simulink model "simulink_2D_Quadrotor_and_pendulum"  (R2023a)
settings: Solver=ode4  StartTime=0.0  StopTime=15  FixedStep=1e-3  RelTol=1e-3
values from neighbouring files (symbols this model uses):
  d = 0.1    [parametry_Lagrange.m]    (also in parametry_a_vizualizace.m)
  g = 9.81    [parametry_Lagrange.m]    (also in parametry_a_vizualizace.m)
  Ikv = 0.00025    [parametry_Lagrange.m]    (also in parametry_a_vizualizace.m)
  Ip = m*d^2    (= 0.0001)    [parametry_Lagrange.m]    (also in parametry_a_vizualizace.m)
  k = 0    [parametry_Lagrange.m]    (also in parametry_a_vizualizace.m = 0.1)
  kp = 0    [parametry_Lagrange.m]    (also in parametry_a_vizualizace.m = 0.01)
  L = 0.086    [parametry_Lagrange.m]    (also in parametry_a_vizualizace.m)
  M = 0.5    [parametry_Lagrange.m]    (also in parametry_a_vizualizace.m)
  m = 0.01    [parametry_Lagrange.m]    (also in parametry_a_vizualizace.m)
libraries: slpidlib x3, simulink_extras x2
settings Model: PacingRate=5  Creator=Admin  LastModifiedBy=Admin

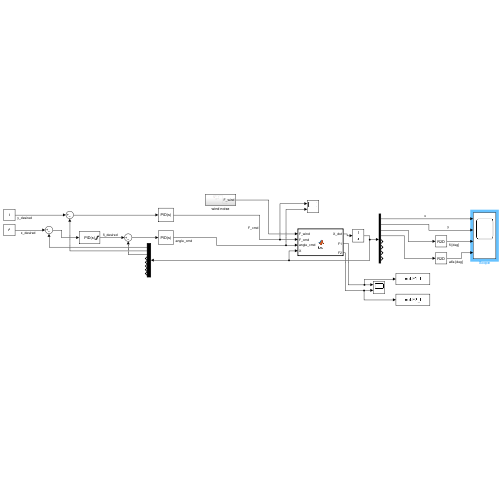
[thumbnail: Simulink's stored preview of the top-level diagram]
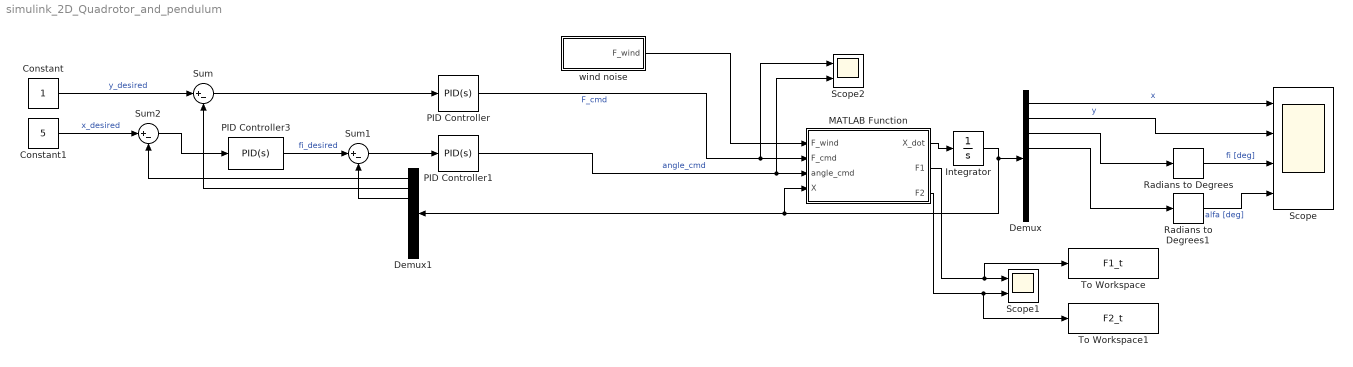
== system simulink_2D_Quadrotor_and_pendulum ==
  Constant : Constant
  Constant1 : Constant  Value=5
  Demux : Demux  Outputs=8
  Demux1 : Demux  Outputs=8
  Integrator : Integrator  InitialCondition=[0;0;0;0;0;0;0;0]  UpperSaturationLimit=[inf; inf; inf; pi; inf; inf; inf; inf]  LowerSaturationLimit=[-inf; -inf; -inf; -pi; -inf; -inf; -inf; -inf]  IgnoreLimit=on
  MATLAB Function : MATLAB Function  TreatAsAtomicUnit=on
  PID Controller : slpidlib/PID Controller  Controller=PID  Form=Parallel  TimeDomain=Continuous-time  UseExternalTs=off  SampleTime=-1  IntegratorMethod=Forward Euler  FilterMethod=Forward Euler  ControllerParametersSource=internal  P=1.05198564586534  I=0.256782152616  UseKiTs=off  D=0.957105978156924  N=439.006628920084  UseFilter=on  TunerSelectOption=Transfer Function Based (PID Tuner App)  InitialConditionSource=internal  InitialConditionForIntegrator=0  InitialConditionForFilter=0  DifferentiatorICPrevScaledInput=0  ExternalReset=none  TrackingMode=off  Kt=1  LimitOutput=off  SatLimitsSource=internal  UpperSaturationLimit=inf  LowerSaturationLimit=-inf  LinearizeAsGain=on  AntiWindupMode=none  Kb=1  LimitIntegrator=off  UpperIntegratorSaturationLimit=inf  LowerIntegratorSaturationLimit=-inf  POutMin=[]  POutMax=[]  IOutMin=[]  IOutMax=[]  DOutMin=[]  DOutMax=[]  NOutMin=[]  NOutMax=[]  SumOutMin=[]  SumOutMax=[]  SaturationOutMin=[]  SaturationOutMax=[]  PParamMin=[]  PParamMax=[]  IParamMin=[]  IParamMax=[]  DParamMin=[]  DParamMax=[]  NParamMin=[]  NParamMax=[]  KbParamMin=[]  KbParamMax=[]  KtParamMin=[]  KtParamMax=[]  KbOutMin=[]  KbOutMax=[]  KtOutMin=[]  KtOutMax=[]  IntegratorOutMin=[]  IntegratorOutMax=[]  FilterOutMin=[]  FilterOutMax=[]  SumI1OutMin=[]  SumI1OutMax=[]  SumI2OutMin=[]  SumI2OutMax=[]  SumI3OutMin=[]  SumI3OutMax=[]  SumI4OutMin=[]  SumI4OutMax=[]  SumDOutMin=[]  SumDOutMax=[]  DifferentiatorOutMin=[]  DifferentiatorOutMax=[]  FilterDiffOutCoefMin=[]  FilterDiffOutCoefMax=[]  ReciprocalOutMin=[]  ReciprocalOutMax=[]  SumDenOutMin=[]  SumDenOutMax=[]  SumNumOutMin=[]  SumNumOutMax=[]  DivideOutMin=[]  DivideOutMax=[]  UdiffTsProdOutMin=[]  UdiffTsProdOutMax=[]  NTsProdOutMin=[]  NTsProdOutMax=[]  UintegralTsProdOutMin=[]  UintegralTsProdOutMax=[]  UngainTsProdOutMin=[]  UngainTsProdOutMax=[]  ClampingZeroOutDataTypeStr=Inherit: Inherit via back propagation  ClampingZeroOutMin=[]  ClampingZeroOutMax=[]  FilterDenConstantOutDataTypeStr=Inherit: Inherit via back propagation  FilterDenConstantOutMin=[]  FilterDenConstantOutMax=[]  PCopyOutDataTypeStr=Inherit: Inherit via back propagation  PCopyOutMin=[]  PCopyOutMax=[]  NCopyOutDataTypeStr=Inherit: Inherit via back propagation  NCopyOutMin=[]  NCopyOutMax=[]  IntegratorContinuousStateAttributes=''  IntegratorStateMustResolveToSignalObject=off  IntegratorRTWStateStorageClass=Auto  FilterContinuousStateAttributes=''  FilterStateMustResolveToSignalObject=off  FilterRTWStateStorageClass=Auto  ParallelPVariant=InternalParameters  IdealPVariant=Disabled  IVariant=InternalParameters  DVariant=InternalParameters  IntegratorVariant=Continuous  SatVariant=Disabled  AWVariant=Passthrough  PCopyVariant=Disabled  TRVariant=Disabled  FdbkBlocksVariant=Forward  IdealPFdbkVariant=Disabled  SatFdbkVariant=Disabled  DerivativeFilterVariant=ContFilter  NVariant=InternalParameters  NCopyVariant=Disabled  FilterICVariant=InternalICsFilter  IntegratorICVariant=InternalICs  ExternalResetVariant=Disabled  TRSumVariant=Passthrough  SumFdbkVariant=Disabled  SumVariant=Sum_PID  TsampFilterVariant=InternalTs  TsampNgainVariant=Passthrough  TsampIntegralVariant=Passthrough  ExternalSaturationOutDataTypeStr=Inherit: Same as second input
  PID Controller1 : slpidlib/PID Controller  Controller=PID  Form=Parallel  TimeDomain=Continuous-time  UseExternalTs=off  SampleTime=-1  IntegratorMethod=Forward Euler  FilterMethod=Forward Euler  ControllerParametersSource=internal  P=0.0094983620396136  I=0.000297296508384773  UseKiTs=off  D=0.00438770568667322  N=3.63078054770101  UseFilter=on  TunerSelectOption=Transfer Function Based (PID Tuner App)  InitialConditionSource=internal  InitialConditionForIntegrator=0  InitialConditionForFilter=0  DifferentiatorICPrevScaledInput=0  ExternalReset=none  TrackingMode=off  Kt=1  LimitOutput=off  SatLimitsSource=internal  UpperSaturationLimit=inf  LowerSaturationLimit=-inf  LinearizeAsGain=on  AntiWindupMode=none  Kb=1  LimitIntegrator=off  UpperIntegratorSaturationLimit=inf  LowerIntegratorSaturationLimit=-inf  POutMin=[]  POutMax=[]  IOutMin=[]  IOutMax=[]  DOutMin=[]  DOutMax=[]  NOutMin=[]  NOutMax=[]  SumOutMin=[]  SumOutMax=[]  SaturationOutMin=[]  SaturationOutMax=[]  PParamMin=[]  PParamMax=[]  IParamMin=[]  IParamMax=[]  DParamMin=[]  DParamMax=[]  NParamMin=[]  NParamMax=[]  KbParamMin=[]  KbParamMax=[]  KtParamMin=[]  KtParamMax=[]  KbOutMin=[]  KbOutMax=[]  KtOutMin=[]  KtOutMax=[]  IntegratorOutMin=[]  IntegratorOutMax=[]  FilterOutMin=[]  FilterOutMax=[]  SumI1OutMin=[]  SumI1OutMax=[]  SumI2OutMin=[]  SumI2OutMax=[]  SumI3OutMin=[]  SumI3OutMax=[]  SumI4OutMin=[]  SumI4OutMax=[]  SumDOutMin=[]  SumDOutMax=[]  DifferentiatorOutMin=[]  DifferentiatorOutMax=[]  FilterDiffOutCoefMin=[]  FilterDiffOutCoefMax=[]  ReciprocalOutMin=[]  ReciprocalOutMax=[]  SumDenOutMin=[]  SumDenOutMax=[]  SumNumOutMin=[]  SumNumOutMax=[]  DivideOutMin=[]  DivideOutMax=[]  UdiffTsProdOutMin=[]  UdiffTsProdOutMax=[]  NTsProdOutMin=[]  NTsProdOutMax=[]  UintegralTsProdOutMin=[]  UintegralTsProdOutMax=[]  UngainTsProdOutMin=[]  UngainTsProdOutMax=[]  ClampingZeroOutDataTypeStr=Inherit: Inherit via back propagation  ClampingZeroOutMin=[]  ClampingZeroOutMax=[]  FilterDenConstantOutDataTypeStr=Inherit: Inherit via back propagation  FilterDenConstantOutMin=[]  FilterDenConstantOutMax=[]  PCopyOutDataTypeStr=Inherit: Inherit via back propagation  PCopyOutMin=[]  PCopyOutMax=[]  NCopyOutDataTypeStr=Inherit: Inherit via back propagation  NCopyOutMin=[]  NCopyOutMax=[]  IntegratorContinuousStateAttributes=''  IntegratorStateMustResolveToSignalObject=off  IntegratorRTWStateStorageClass=Auto  FilterContinuousStateAttributes=''  FilterStateMustResolveToSignalObject=off  FilterRTWStateStorageClass=Auto  ParallelPVariant=InternalParameters  IdealPVariant=Disabled  IVariant=InternalParameters  DVariant=InternalParameters  IntegratorVariant=Continuous  SatVariant=Disabled  AWVariant=Passthrough  PCopyVariant=Disabled  TRVariant=Disabled  FdbkBlocksVariant=Forward  IdealPFdbkVariant=Disabled  SatFdbkVariant=Disabled  DerivativeFilterVariant=ContFilter  NVariant=InternalParameters  NCopyVariant=Disabled  FilterICVariant=InternalICsFilter  IntegratorICVariant=InternalICs  ExternalResetVariant=Disabled  TRSumVariant=Passthrough  SumFdbkVariant=Disabled  SumVariant=Sum_PID  TsampFilterVariant=InternalTs  TsampNgainVariant=Passthrough  TsampIntegralVariant=Passthrough  ExternalSaturationOutDataTypeStr=Inherit: Same as second input
  PID Controller3 : slpidlib/PID Controller  Controller=PID  Form=Parallel  TimeDomain=Continuous-time  UseExternalTs=off  SampleTime=-1  IntegratorMethod=Forward Euler  FilterMethod=Forward Euler  ControllerParametersSource=internal  P=-0.0116363168342293  I=-6.9932407082639e-05  UseKiTs=off  D=-0.0557959195476428  N=0.708041105970502  UseFilter=on  TunerSelectOption=Transfer Function Based (PID Tuner App)  InitialConditionSource=internal  InitialConditionForIntegrator=0  InitialConditionForFilter=0  DifferentiatorICPrevScaledInput=0  ExternalReset=none  TrackingMode=off  Kt=1  LimitOutput=on  SatLimitsSource=internal  UpperSaturationLimit=pi/2  LowerSaturationLimit=-pi/2  LinearizeAsGain=off  AntiWindupMode=none  Kb=1  LimitIntegrator=off  UpperIntegratorSaturationLimit=inf  LowerIntegratorSaturationLimit=-inf  POutMin=[]  POutMax=[]  IOutMin=[]  IOutMax=[]  DOutMin=[]  DOutMax=[]  NOutMin=[]  NOutMax=[]  SumOutMin=[]  SumOutMax=[]  SaturationOutMin=[]  SaturationOutMax=[]  PParamMin=[]  PParamMax=[]  IParamMin=[]  IParamMax=[]  DParamMin=[]  DParamMax=[]  NParamMin=[]  NParamMax=[]  KbParamMin=[]  KbParamMax=[]  KtParamMin=[]  KtParamMax=[]  KbOutMin=[]  KbOutMax=[]  KtOutMin=[]  KtOutMax=[]  IntegratorOutMin=[]  IntegratorOutMax=[]  FilterOutMin=[]  FilterOutMax=[]  SumI1OutMin=[]  SumI1OutMax=[]  SumI2OutMin=[]  SumI2OutMax=[]  SumI3OutMin=[]  SumI3OutMax=[]  SumI4OutMin=[]  SumI4OutMax=[]  SumDOutMin=[]  SumDOutMax=[]  DifferentiatorOutMin=[]  DifferentiatorOutMax=[]  FilterDiffOutCoefMin=[]  FilterDiffOutCoefMax=[]  ReciprocalOutMin=[]  ReciprocalOutMax=[]  SumDenOutMin=[]  SumDenOutMax=[]  SumNumOutMin=[]  SumNumOutMax=[]  DivideOutMin=[]  DivideOutMax=[]  UdiffTsProdOutMin=[]  UdiffTsProdOutMax=[]  NTsProdOutMin=[]  NTsProdOutMax=[]  UintegralTsProdOutMin=[]  UintegralTsProdOutMax=[]  UngainTsProdOutMin=[]  UngainTsProdOutMax=[]  ClampingZeroOutDataTypeStr=Inherit: Inherit via back propagation  ClampingZeroOutMin=[]  ClampingZeroOutMax=[]  FilterDenConstantOutDataTypeStr=Inherit: Inherit via back propagation  FilterDenConstantOutMin=[]  FilterDenConstantOutMax=[]  PCopyOutDataTypeStr=Inherit: Inherit via back propagation  PCopyOutMin=[]  PCopyOutMax=[]  NCopyOutDataTypeStr=Inherit: Inherit via back propagation  NCopyOutMin=[]  NCopyOutMax=[]  IntegratorContinuousStateAttributes=''  IntegratorStateMustResolveToSignalObject=off  IntegratorRTWStateStorageClass=Auto  FilterContinuousStateAttributes=''  FilterStateMustResolveToSignalObject=off  FilterRTWStateStorageClass=Auto  ParallelPVariant=InternalParameters  IdealPVariant=Disabled  IVariant=InternalParameters  DVariant=InternalParameters  IntegratorVariant=Continuous  SatVariant=Disabled  AWVariant=Passthrough  PCopyVariant=Disabled  TRVariant=Disabled  FdbkBlocksVariant=Forward  IdealPFdbkVariant=Disabled  SatFdbkVariant=Disabled  DerivativeFilterVariant=ContFilter  NVariant=InternalParameters  NCopyVariant=Disabled  FilterICVariant=InternalICsFilter  IntegratorICVariant=InternalICs  ExternalResetVariant=Disabled  TRSumVariant=Passthrough  SumFdbkVariant=Disabled  SumVariant=Sum_PID  TsampFilterVariant=InternalTs  TsampNgainVariant=Passthrough  TsampIntegralVariant=Passthrough  ExternalSaturationOutDataTypeStr=Inherit: Same as second input
  Radians to Degrees : simulink_extras/Transformations/Radians to Degrees
  Radians to Degrees1 : simulink_extras/Transformations/Radians to Degrees
  Scope : Scope  NumInputPorts=4
  Scope1 : Scope  NumInputPorts=2
  Scope2 : Scope  NumInputPorts=2
  Sum : Sum  Inputs=|+-
  Sum1 : Sum  Inputs=|+-
  Sum2 : Sum  Inputs=|+-
  To Workspace : ToWorkspace  VariableName=F1_t  SampleTime=-1
  To Workspace1 : ToWorkspace  VariableName=F2_t  SampleTime=-1
  wind noise : Subsystem
  wires:
  MATLAB Function/1(X_dot) -> Integrator/1
  Integrator/1 -> Demux1/1, MATLAB Function/4(X), Demux/1
  Demux/3 -> Radians to Degrees/1
  Demux/2 -> Scope/2  "y"
  Demux/1 -> Scope/1  "x"
  PID Controller/1 -> Scope2/1, MATLAB Function/2(F_cmd)  "F_cmd"
  PID Controller1/1 -> Scope2/2, MATLAB Function/3(angle_cmd)  "angle_cmd"
  Constant/1 -> Sum/1  "y_desired"
  Sum/1 -> PID Controller/1
  PID Controller3/1 -> Sum1/1  "fi_desired"
  Sum1/1 -> PID Controller1/1
  Constant1/1 -> Sum2/1  "x_desired"
  Sum2/1 -> PID Controller3/1
  Radians to Degrees/1 -> Scope/3  "fi [deg]"
  Demux/4 -> Radians to Degrees1/1
  Radians to Degrees1/1 -> Scope/4  "alfa [deg]"
  wind noise/1(F_wind) -> MATLAB Function/1(F_wind)
  Demux1/2 -> Sum/2
  Demux1/3 -> Sum1/2
  Demux1/1 -> Sum2/2
  MATLAB Function/2(F1) -> To Workspace/1, Scope1/1
  MATLAB Function/3(F2) -> To Workspace1/1, Scope1/2

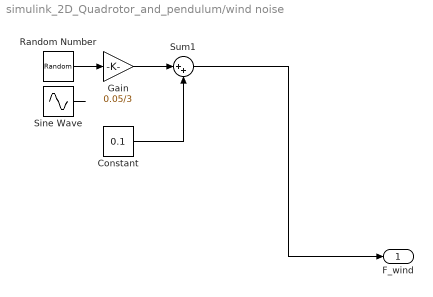
== system simulink_2D_Quadrotor_and_pendulum/wind noise ==
  Constant : Constant  Value=0.1
  Gain : Gain  Gain=0.05/3
  Random Number : RandomNumber  SampleTime=0.1
  Sine Wave : Sin  Amplitude=0.1  Frequency=0.5  SampleTime=0
  Sum1 : Sum  Inputs=|++
  F_wind : Outport
  wires:
  Sum1/1 -> F_wind/1
  Gain/1 -> Sum1/1
  Sine Wave/1 -> ?
  Random Number/1 -> Gain/1
  Constant/1 -> Sum1/2

== matlab function simulink_2D_Quadrotor_and_pendulum/MATLAB Function ==
  data: F_wind input; F_cmd input; angle_cmd input; X_dot output; X input; g parameter; L parameter; d parameter; M parameter; m parameter; Ikv parameter; Ip parameter; k parameter; kp parameter; F1 output; F2 output
function [X_dot, F1, F2]= fcn(F_wind, F_cmd, angle_cmd, X, g, L, d, M, m, Ikv, Ip, k, kp)
% [x1, x2, x3, x4, x5, x6, x7, x8] = [x, y, fi, alfa, x_dot, y_dot, fi_dot, alfa_dot]
x1 = X(1);
x2 = X(2);
x3 = X(3);
x4 = X(4);
x5 = X(5);
x6 = X(6);
x7 = X(7);
x8 = X(8);

F1 = F_cmd + angle_cmd; % Celková tažná síla na 1. motoru
F2 = F_cmd - angle_cmd; % Celková tažná síla na 2. motoru
% F1 a F2 lze také vyjádřit přes úhlové rychlosti motorů, např.
% w1 = F_cmd + angle_cmd
% w2 = F_cmd - angle_cmd
% F1 = koef * w1^2; F2 = koef * w2^2


x1_dot = x5;
x2_dot = x6;
x3_dot = x7;
x4_dot = x8;

x5_dot = -(sin(x3)*(F1 + F2) - F_wind - m*(d*x8^2*sin(x4) - g*cos(x4)*sin(x4)) + k*x5 + kp*(x5 + d*x8*cos(x4)))/(M + m);
x6_dot = -(M*g - cos(x3)*(F1 + F2) + g*m + k*x6 + m*(d*cos(x4)*x8^2 + g*sin(x4)^2) + kp*(x6 + d*x8*sin(x4)))/(M + m);
x7_dot = (F1-F2)*L/Ikv;

x8_dot = -(kp*x5*cos(x4) + g*m*sin(x4) + kp*x6*sin(x4) + d*kp*x8 - (m*cos(x4)*(sin(x3)*(F1 + F2) - F_wind - m*(d*x8^2*sin(x4) - g*cos(x4)*sin(x4)) + k*x5 + kp*(x5 + d*x8*cos(x4))))/(M + m) - (m*sin(x4)*(M*g - cos(x3)*(F1 + F2) + g*m + k*x6 + m*(d*cos(x4)*x8^2 + g*sin(x4)^2) + kp*(x6 + d*x8*sin(x4))))/(M + m))/(d*m);

X_dot = [x1_dot, x2_dot, x3_dot, x4_dot, x5_dot, x6_dot, x7_dot, x8_dot]';
